simulink model "SqWv_Without_SG"  (R2025b)
settings: Solver=FixedStepDiscrete  StartTime=0.0  StopTime=0.1  FixedStep=0.01  RelTol=1e-3
settings Model: Creator=soura  LastModifiedBy=soura

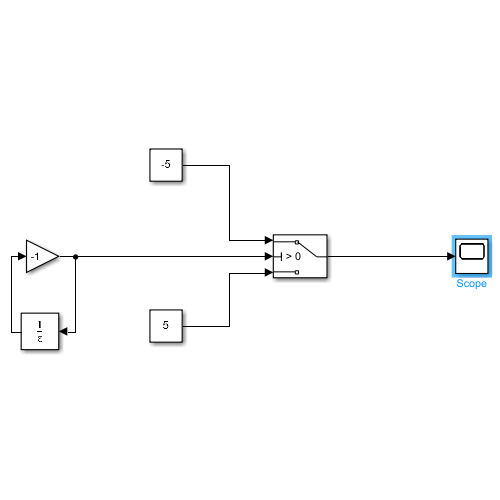
[thumbnail: Simulink's stored preview of the top-level diagram]
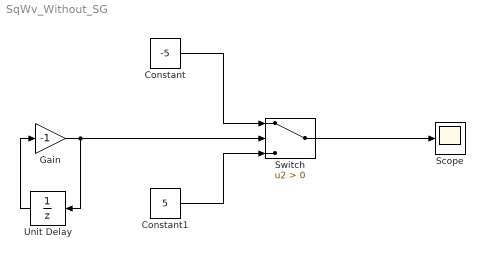
== system SqWv_Without_SG ==
  Constant : Constant  Value=-5
  Constant1 : Constant  Value=5
  Gain : Gain  Gain=-1
  Scope : Scope
      settings: ActiveDisplayYMinimum=-6.25  ActiveDisplayYMaximum=6.25
  Switch : Switch  Criteria=u2 > Threshold  SaturateOnIntegerOverflow=off  InputSameDT=off
  Unit Delay : UnitDelay  InitialCondition=1  SampleTime=-1  HasFrameUpgradeWarning=on
  wires:
  Unit Delay/1 -> Gain/1
  Gain/1 -> Switch/2, Unit Delay/1
  Constant/1 -> Switch/1
  Constant1/1 -> Switch/3
  Switch/1 -> Scope/1
